simulink model "ECE551_proj1_2017"  (R2017b)
settings: Solver=VariableStepAuto  StartTime=0.0  StopTime=0.03  RelTol=1e-3
values from neighbouring files (symbols this model uses):
  A = d*A1+d1*A2    [269_1.m]    (also in DifRelFil.m = (2/Nsc)*cos(2*pi*n/Nsc); DigiDiffRelay.m = (2/Nsc)*cos(2*pi*n/Nsc); DigiRelay.m = (2/Nsc)*cos(2*pi*n/Nsc); DigiRelay2.m = (2/Nsc)*cos(2*pi*n/Nsc))
  B = d*B1+d1*B2    [269_1.m]    (also in DifRelFil.m = (2/Nsc)*sin(2*pi*n/Nsc); DigiDiffRelay.m = (2/Nsc)*sin(2*pi*n/Nsc); DigiRelay.m = (2/Nsc)*sin(2*pi*n/Nsc); DigiRelay2.m = (2/Nsc)*sin(2*pi*n/Nsc))
  Bd = (A1−A2)*X    [269_1.m]    (also in ECE551_Project_part1.m = (A1-A2)*X; ECE551_Project_part2.m = (A1-A2)*X)
  C = d*C1+d1*C2    [269_1.m]    (also in ECE347HW5.m = Yc*(1 + Z*Yc/4); ECE545HW6.m = 0.001; ECE551HW1.m = 0.0001; ECE551_Project_part1.m)
settings Model: Creator=clarke6  LastModifiedBy=clarke6

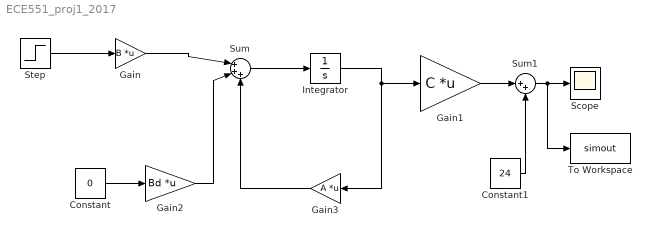
== system ECE551_proj1_2017 ==
  Constant : Constant  Value=0
  Constant1 : Constant  Value=24
  Gain : Gain  Gain=B  Multiplication=Matrix(K*u)
  Gain1 : Gain  Gain=C  Multiplication=Matrix(K*u)
  Gain2 : Gain  Gain=Bd  Multiplication=Matrix(K*u)
  Gain3 : Gain  Gain=A  Multiplication=Matrix(K*u)
  Integrator : Integrator
  Scope : Scope
  Step : Step  Time=0  SampleTime=0
  Sum : Sum  Inputs=|+++
  Sum1 : Sum  Inputs=|++
  To Workspace : ToWorkspace  VariableName=simout  SaveFormat=Timeseries  SampleTime=-1
  wires:
  Gain/1 -> Sum/1
  Gain2/1 -> Sum/2
  Gain3/1 -> Sum/3
  Sum/1 -> Integrator/1
  Integrator/1 -> Gain3/1, Gain1/1
  Step/1 -> Gain/1
  Sum1/1 -> To Workspace/1, Scope/1
  Gain1/1 -> Sum1/1
  Constant/1 -> Gain2/1
  Constant1/1 -> Sum1/2
